simulink model "model2"  (R2016a)
settings: Solver=VariableStepAuto  StartTime=0.0  StopTime=10.0  RelTol=1e-3
values from neighbouring files (symbols this model uses):
  b = 0.7    [main.m]
  Fe = 10    [main.m]
  k = 5    [main.m]
  l10 = 1    [main.m]
  M = 2    [main.m]
  m = 10    [main.m]
  y0 = 2*l10    (= 2)    [main.m]    (also in model2sim.m = ic(3))
settings Model: Creator=marek  LastModifiedBy=marek
settings GRTTargetCC: GeneratePreprocessorConditionals=Use local settings

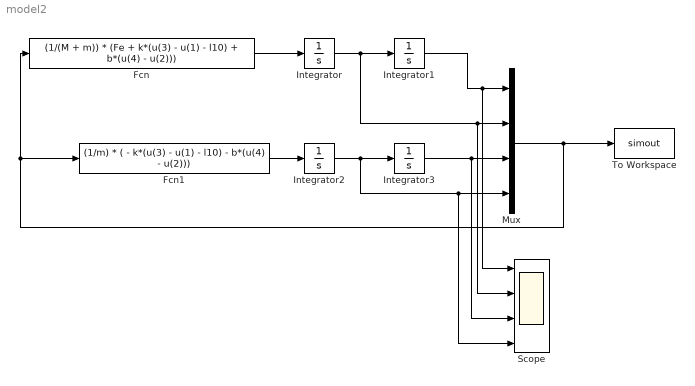
== system model2 ==
  Fcn : Fcn  Expr=(1/(M + m)) * (Fe + k*(u(3) - u(1) - l10) + b*(u(4) - u(2)))
  Fcn1 : Fcn  Expr=(1/m) * ( - k*(u(3) - u(1) - l10) - b*(u(4) - u(2)))
  Integrator : Integrator
  Integrator1 : Integrator
  Integrator2 : Integrator
  Integrator3 : Integrator  InitialCondition=y0
  Mux : Mux
  Scope : Scope  NumInputPorts=4
  To Workspace : ToWorkspace  VariableName=simout  SampleTime=-1
  wires:
  Integrator/1 -> Scope/2, Mux/2, Integrator1/1
  Integrator1/1 -> Scope/1, Mux/1
  Integrator2/1 -> Scope/4, Mux/4, Integrator3/1
  Integrator3/1 -> Scope/3, Mux/3
  Mux/1 -> Fcn1/1, Fcn/1, To Workspace/1
  Fcn/1 -> Integrator/1
  Fcn1/1 -> Integrator2/1
